simulink model "w13"  (R2025a)
settings: Solver=VariableStepAuto  StartTime=0.0  StopTime=3  FixedStep=1e-5  MaxStep=1e-4  RelTol=1e-3
values from neighbouring files (symbols this model uses):
  B = 0.0001    [main.m]
  Is_rated = 10    [main.m]
  J = 0.045    [main.m]
  Kas = 1/Kps    (= 3.05577490736)    [main.m]
  Kic = Rs*Wcc    (= 1256.63706144)    [main.m]
  Kis = J*Wsc^2/5/Kt    (= 2.05616758356)    [main.m]
  Kpc = Lds*Wcc    (= 18.8495559215)    [main.m]
  Kps = J*Wsc/Kt    (= 0.327249234749)    [main.m]
  Lamf = 0.12    [main.m]
  Lds = 30.0e-3    (= 0.03)    [main.m]
  Lqs = 40.0e-3    (= 0.04)    [main.m]
  P = 24    [main.m]
  Rs = 2    [main.m]
  Wcc = 100*2*pi    (= 628.318530718)    [main.m]
settings Model: Creator=moon  LastModifiedBy=New
settings RTWCC: GPUComputeCapability=3.5

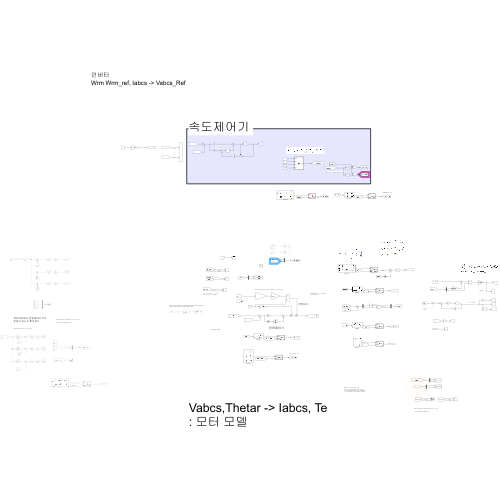
[thumbnail: Simulink's stored preview of the top-level diagram]
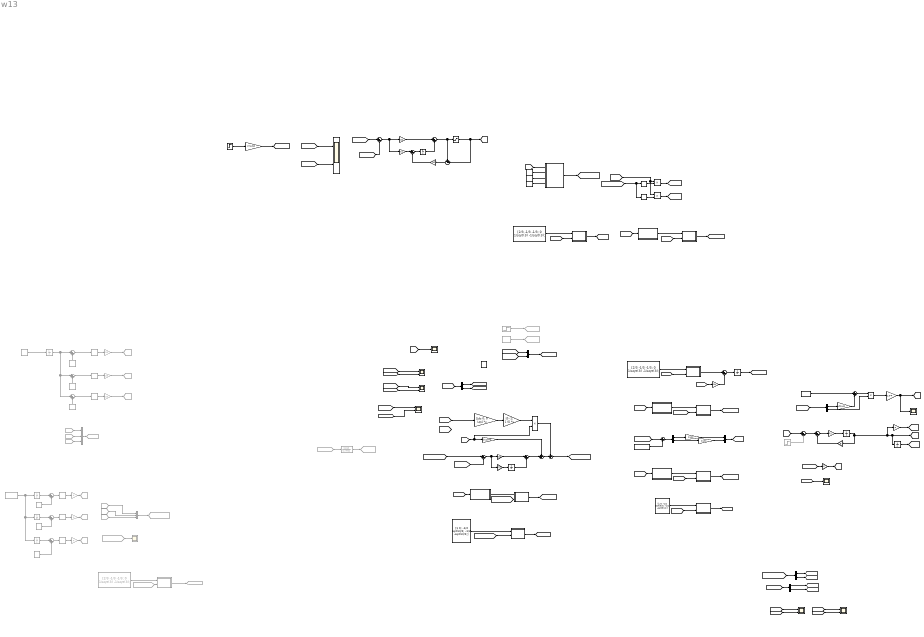
== system w13 ==
  note: 30도 더하면 속도제어가 안정적이게 된다
  note: E = w*phi 라서 속도는 전압에 비례
      | T는 전류에 비례
  note: 인버터
      | Wrm Wrm_ref, Iabcs -> Vabcs_Ref
  note: 전류제어기
  note: Vabcs,Thetar -> Iabcs, Te
      | : 모터 모델
  note: 컴퓨터에서 사용하는 값. 센싱된것. Idqsr과 무슨 차이? 센싱만?
  note: 센싱된 것을 사용해야
  note: 여기 수정함
  note: 여기서 부터는 모터
  note: 두개를 비교해보면 똑같을 것. 실제에 LPF를 넣을 순없다. LPF는 이상적인 상황. 이론적으로 실제 전류는 LPF와 이론적으로 같을 것이다
  note: feedback 이라는 뜻
  note: 속도제어기
  note: +였나?
  note: 전향보상
  note: 4Nm 만큼 거리가 발생해서 회전,
      | 외부 토크가 발생해도iqs 만큼 무조건 제어
      | 그럼 어떻게 회전자계와 회전자의 위치를 맞춰?
      | -> 기계 모델링을 무시: 대신 "wrm이 고정이다"
  note: d축과 q축 에 대한 정보가 아무 것도 없다
  note: 그래서 동기좌표 제어를 해야한다
  note: Wcc 와 We의 차이 만큼 딜레이와 크기 차이가 발생
  note: 정지좌표에서 전류제어기 무슨 문제가 있는지 확인한다
  note: 1/2 해야?
  note: Wcc 와 We의 차이 만큼 딜레이와 크기 차이가 발생
  note: 그래서 동기좌표 제어를 해야한다
  Constant : Constant  Commented=on  Value=10
  Constant1 : Constant  Commented=on  Value=2*pi/3
  Constant10 : Constant  Commented=on  Value=4
  Constant11 : Constant  Commented=on  Value=-4*pi/3
  Constant13 : Constant  Value=Lds
  Constant14 : Constant  Value=Lqs
  Constant15 : Constant  Value=Lamf
  Constant2 : Constant  Commented=on  Value=-2*pi/3
  Constant3 : Constant  Value=[Lamf 0 ]
  Constant4 : Constant  Value=Lamf
  Constant5 : Constant  Commented=on  Value=0
  Constant6 : Constant  Commented=on  Value=10*2*pi
  Constant7 : Constant  Commented=on  Value=0
  Constant8 : Constant  Value=0
  Constant9 : Constant  Commented=on  Value=-2*pi/3
  Cos : Trigonometry  Commented=on  Operator=cos
  Cos1 : Trigonometry  Commented=on  Operator=cos
  Cos2 : Trigonometry  Commented=on  Operator=cos
  Cos3 : Trigonometry  Operator=cos
  Demux{,1..2,4..5} (5 alike) : Demux  Outputs=2
  From18 : From  Commented=on  GotoTag=Vas
  From19 : From  Commented=on  GotoTag=Vbs
  From2 : From  Commented=on  GotoTag=Iabcs_Ref
  From20 : From  Commented=on  GotoTag=Vcs
  From22 : From  Commented=on  GotoTag=Ias_Ref
  From23 : From  Commented=on  GotoTag=Ibs_Ref
  From24 : From  Commented=on  GotoTag=Ics_Ref
  From26 : From  Commented=on  GotoTag=Iabcs_Ref
  From53 : From  Commented=on  GotoTag=Idqsr_Ref
  Gain : Gain  Commented=on  Gain=20
  Gain1 : Gain  Commented=on  Gain=20
  Gain10 : Gain  Gain=1/Lds
  Gain11 : Gain  Gain=1/Lqs
  Gain12 : Gain  Gain=[0 Lamf]
  Gain13 : Gain  Gain=[Lds 0; 0 Lqs]  Multiplication=Matrix(K*u)
  Gain14 : Gain  Gain=Kps
  Gain15 : Gain  Gain=Kis
  Gain16 : Gain  Gain=Kas
  Gain17 : Gain  Gain=2*pi/60
  Gain19 : Gain  Gain=Lds-Lqs
  Gain2 : Gain  Commented=on  Gain=20
  Gain20 : Gain  Gain=1.5*P
  Gain21 : Gain  Gain=Rs
  Gain22 : Gain  Gain=P
  Gain23 : Gain  Gain=1/J
  Gain24 : Gain  Gain=B
  Gain3 : Gain  Commented=on  Gain=4
  Gain4 : Gain  Commented=on  Gain=4
  Gain5 : Gain  Commented=on  Gain=4
  Gain6 : Gain  Gain=Kpc
  Gain7 : Gain  Gain=Kic
  Gain8 : Gain  Gain=[0 -1; 1 0]  Multiplication=Matrix(K*u)
  Gain9 : Gain  Gain=P
  Goto : Goto  Commented=on  GotoTag=Vas
  Goto1 : Goto  Commented=on  GotoTag=Vbs
  Goto14 : Goto  Commented=on  GotoTag=Ibs_Ref
  Goto15 : Goto  Commented=on  GotoTag=Ics_Ref
  Goto16 : Goto  Commented=on  GotoTag=Iabcs_Ref
  Goto17 : Goto  Commented=on  GotoTag=Idqss_Ref
  Goto18 : Goto  Commented=on  GotoTag=Idsr_Ref
  Goto19 : Goto  Commented=on  GotoTag=Iqsr_Ref
  Goto2 : Goto  Commented=on  GotoTag=Vcs
  Goto38 : Goto  Commented=on  GotoTag=Idqsr_FB
  Goto4 : Goto  Commented=on  GotoTag=Vabcs
  Goto9 : Goto  Commented=on  GotoTag=Ias_Ref
  Integrator{,4..6} (4 alike) : Integrator  Commented=on
  Integrator{1..3,7..8} (5 alike) : Integrator
  MATLAB Function : MATLAB Function  TreatAsAtomicUnit=on
  MATLAB Function1 : MATLAB Function  TreatAsAtomicUnit=on
  MATLAB Function2 : MATLAB Function  TreatAsAtomicUnit=on
  MATLAB Function3 : MATLAB Function  TreatAsAtomicUnit=on
  MATLAB Function4 : MATLAB Function  Commented=on  TreatAsAtomicUnit=on
  MATLAB Function5 : MATLAB Function  TreatAsAtomicUnit=on
  MATLAB Function6 : MATLAB Function  TreatAsAtomicUnit=on
  MATLAB Function7 : MATLAB Function  TreatAsAtomicUnit=on
  MATLAB Function8 : MATLAB Function  TreatAsAtomicUnit=on
  MATLAB Function9 : MATLAB Function  TreatAsAtomicUnit=on
  Mux : Mux  Commented=on  Inputs=3
  Mux1 : Mux  Commented=on  Inputs=3
  Mux2 : Mux  Inputs=2
  Mux3 : Mux  Inputs=2
  Product{,1..2,8} (4 alike) : Product
  R(-theta) : Subsystem
      mask Display: image(imread('img/rotateInverseMatrix.png'))
  R(-theta)1 : Subsystem
      mask Display: image(imread('img/rotateInverseMatrix.png'))
  R(theta) : Subsystem
      mask Display: image(imread('img/rotateMatrix.png'))
  R(theta)1 : Subsystem
      mask Display: image(imread('img/rotateMatrix.png'))
  Saturation : Saturate  UpperLimit=Is_rated  LowerLimit=-Is_rated
  Scope : Scope
      settings: ActiveDisplayYMinimum=-12.65498  ActiveDisplayYMaximum=12.66704
  Scope1 : Scope  Commented=on
      settings: ActiveDisplayYMinimum=-5  ActiveDisplayYMaximum=5
  Scope2 : Scope
      settings: ActiveDisplayYMinimum=-30.63126  ActiveDisplayYMaximum=63.40805  DataLoggingVariableName=ScopeData2
  Scope{3..8} (6 alike) : Scope  NumInputPorts=2
      Scope3 settings: ActiveDisplayYMinimum=-5.30172  ActiveDisplayYMaximum=0.86593  DataLoggingVariableName=ScopeData4
      Scope4 settings: ActiveDisplayYMinimum=-5.10751  ActiveDisplayYMaximum=5.1663  DataLoggingVariableName=ScopeData2
      Scope5 settings: ActiveDisplayYMinimum=-5.08231  ActiveDisplayYMaximum=5.15483  DataLoggingVariableName=ScopeData3
      Scope6 settings: ActiveDisplayYMinimum=-0.50888  ActiveDisplayYMaximum=4.57994  DataLoggingVariableName=ScopeData5
      Scope7 settings: ActiveDisplayYMinimum=-5.25048  ActiveDisplayYMaximum=7.25433  DataLoggingVariableName=ScopeData6
      Scope8 settings: ActiveDisplayYMinimum=-64.34522  ActiveDisplayYMaximum=579.10702
  Scope9 : Scope
      settings: ActiveDisplayYMinimum=-12.65498  ActiveDisplayYMaximum=12.66704
  Sin : Trigonometry  Commented=on
  Sin1 : Trigonometry  Commented=on
  Sin2 : Trigonometry  Commented=on
  Sin3 : Trigonometry
  Step : Step  After=4000  SampleTime=0
  Sum{,1..2,8..10} (6 alike) : Sum  Commented=on  Inputs=|++
  Sum{3..4,6..7,11,15,17} (7 alike) : Sum  Inputs=|+-
  Sum12 : Sum  Inputs=|++
  Sum13 : Sum  Inputs=++|
  Sum14 : Sum  Inputs=++|
  Sum16 : Sum  Inputs=|++
  Sum18 : Sum  Inputs=+-|
  Sum5 : Sum  Inputs=|++
  TL : Step  Commented=on  Time=0.5  SampleTime=0
  Transfer Fcn : TransferFcn  Commented=on  Numerator=[Wcc]  Denominator=[1 Wcc]
  abc to dq : Constant  Value=[2/3 -1/3 -1/3; 0 1/sqrt(3) -1/sqrt(3);]
      mask Display: image(imread('img/abc2dq.png'))
  abc to dq1 : Constant  Commented=on  Value=[2/3 -1/3 -1/3; 0 1/sqrt(3) -1/sqrt(3);]
      mask Display: image(imread('img/abc2dq.png'))
  abc to dq2 : Constant  Value=[2/3 -1/3 -1/3; 0 1/sqrt(3) -1/sqrt(3);]
      mask Display: image(imread('img/abc2dq.png'))
  "at 2s , 4A" : Step  Commented=on  Time=2  After=4  SampleTime=0
  dq to abc : Constant  Value=[1 0; -1/2 sqrt(3)/2; -1/2 -sqrt(3)/2;]
      mask Display: image(imread('img/dq2abc.png'))
  dq to abc1 : Constant  Value=[1 0; -1/2 sqrt(3)/2; -1/2 -sqrt(3)/2;]
      mask Display: image(imread('img/dq2abc.png'))
  wires:
  Gain/1 -> Goto/1
  Sin/1 -> Gain/1
  Sum/1 -> Sin/1
  Constant/1 -> Integrator/1  "angluar velocity"
  Sin1/1 -> Gain1/1
  Gain1/1 -> Goto1/1
  Sum1/1 -> Sin1/1
  Gain2/1 -> Goto2/1
  Sum2/1 -> Sin2/1
  Sin2/1 -> Gain2/1
  Integrator/1 -> Sum2/1, Sum1/1, Sum/1  "angle"
  Constant1/1 -> Sum1/2
  Constant2/1 -> Sum2/2
  Sum3/1 -> Integrator1/1
  Integrator1/1 -> [Lamdqss]
  MATLAB Function3/1(output) -> Sum3/1  "Vdqss"
  [Lamdqsr] -> Sum4/1
  Constant3/1 -> Sum4/2
  Sum4/1 -> Demux1/1
  Demux1/1 -> Gain10/1
  Demux1/2 -> Gain11/1
  Gain10/1 -> Mux2/1
  Gain11/1 -> Mux2/2
  Mux2/1 -> [Idqsr]
  [Idqsr] -> Demux4/1
  Demux4/1 -> Gain19/1
  Constant4/1 -> Sum5/1
  Gain19/1 -> Sum5/2
  Sum5/1 -> Product8/1
  Demux4/2 -> Product8/2
  Product8/1 -> Gain20/1
  Gain20/1 -> Scope2/1, [Te]
  [Te] -> Sum6/1
  Sum6/1 -> Sum7/1
  Integrator3/1 -> Gain24/1, Gain9/1, Integrator2/1, [Wrm]
  TL/1 -> Sum6/2
  [Idqss] -> Gain21/1
  Gain21/1 -> Sum3/2
  Gain22/1 -> [Thetar]
  [Thetarm] -> Gain22/1
  Integrator2/1 -> [Thetarm]
  Sum7/1 -> Gain23/1
  Gain23/1 -> Integrator3/1
  Gain24/1 -> Sum7/2
  dq to abc/1 -> MATLAB Function/1(input1)
  [Idqss] -> MATLAB Function/2(input2)
  MATLAB Function/1(output) -> [Iabcs]
  [Lamdqss] -> MATLAB Function1/2(input2)
  MATLAB Function1/1(output) -> [Lamdqsr]
  [Thetar] -> R(-theta)/1(t)
  R(-theta)/1(y) -> MATLAB Function1/1(input1)
  MATLAB Function2/1(output) -> [Idqss]
  [Thetar] -> R(theta)/1(t)
  R(theta)/1(y) -> MATLAB Function2/1(input1)
  [Idqsr] -> MATLAB Function2/2(input2)
  abc to dq/1 -> MATLAB Function3/1(input1)
  [Vabcs] -> MATLAB Function3/2(input2)
  From18/1 -> Mux1/1
  From19/1 -> Mux1/2
  From20/1 -> Mux1/3
  Mux1/1 -> Goto4/1
  [Iabcs] -> Scope/1
  Constant5/1 -> Sum/2
  Cos/1 -> Gain3/1
  Integrator4/1 -> Sum8/1  "angle"
  Constant7/1 -> Sum8/2
  Sum8/1 -> Cos/1
  Gain3/1 -> Goto9/1
  Gain4/1 -> Goto14/1
  Constant9/1 -> Sum9/2
  Integrator5/1 -> Sum9/1  "angle"
  Sum9/1 -> Cos1/1
  Cos1/1 -> Gain4/1
  Gain5/1 -> Goto15/1
  Constant11/1 -> Sum10/2
  Integrator6/1 -> Sum10/1  "angle"
  Sum10/1 -> Cos2/1
  Cos2/1 -> Gain5/1
  Constant6/1 -> Integrator6/1, Integrator5/1, Integrator4/1  "angluar velocity"
  From22/1 -> Mux/1
  From23/1 -> Mux/2
  From24/1 -> Mux/3
  Mux/1 -> Goto16/1
  MATLAB Function4/1(output) -> Goto17/1
  abc to dq1/1 -> MATLAB Function4/1(input1)
  From26/1 -> MATLAB Function4/2(input2)
  Gain6/1 -> Sum12/1
  Sum11/1 -> Gain7/1, Gain6/1
  Gain7/1 -> Integrator7/1
  Integrator7/1 -> Sum12/2
  dq to abc1/1 -> MATLAB Function5/1(input1)
  MATLAB Function5/1(output) -> [Vabcs]
  [Vdqss_Ref] -> MATLAB Function5/2(input2)
  Demux2/2 -> [Iqs_Ref]
  Demux2/1 -> [Ids_Ref]
  [Idqss_Ref] -> Demux2/1
  [Idqss] -> Demux5/1
  Demux5/1 -> [Idss]
  Demux5/2 -> [Iqss]
  [Ids_Ref] -> Scope4/1  "Ids_Ref"
  [Idss] -> Scope4/2  "Ids"
  [Iqss] -> Scope5/2  "Iqs"
  [Iqs_Ref] -> Scope5/1  "Iqs_Ref"
  From2/1 -> Scope1/1
  "at 2s , 4A"/1 -> Goto18/1
  Constant10/1 -> Goto19/1
  [Iqsr_Ref] -> Mux3/2
  [Idsr_Ref] -> Mux3/1
  Mux3/1 -> [Idqsr_Ref]
  MATLAB Function6/1(output) -> [Vdqss_Ref]
  R(theta)1/1(y) -> MATLAB Function6/1(input1)
  [Vdqsr_Ref] -> MATLAB Function6/2(input2)
  [Thetar] -> R(theta)1/1(t)
  [Idqsr] -> Demux/1
  Demux/2 -> [Iqsr]
  Demux/1 -> [Idsr]
  [Idsr_Ref] -> Scope3/1  "Idsr_Ref"
  [Idsr] -> Scope3/2  "Idsr"
  [Iqsr] -> Scope6/2
  [Iqsr_Ref] -> Scope6/1
  Sum12/1 -> Sum13/2
  Gain9/1 -> [Wr]
  [Wr] -> Product/2, Gain12/1
  Gain12/1 -> Sum13/1
  Sum13/1 -> Sum14/2
  Sum14/1 -> [Vdqsr_Ref]
  [Idqsr] -> Gain13/1
  Gain13/1 -> Gain8/1
  Gain8/1 -> Product/1
  Product/1 -> Sum14/1
  [Idqsr_Ref] -> Scope7/1  "Idqsr_Ref"
  [Idqsr] -> Scope7/2  "Idqsr"
  [Wrm_Ref] -> Sum15/1
  [Wrm] -> Sum15/2
  Gain14/1 -> Sum16/1
  Integrator8/1 -> Sum16/2
  Sum15/1 -> Gain15/1, Gain14/1
  Gain15/1 -> Sum17/1
  Sum17/1 -> Integrator8/1
  Sum16/1 -> Saturation/1, Sum18/1
  Saturation/1 -> [Is_Ref], Sum18/2
  Sum18/1 -> Gain16/1
  Gain16/1 -> Sum17/2
  [Is_Ref] -> MATLAB Function7/1(Is_Ref)
  Constant15/1 -> MATLAB Function7/4(Lamf)
  Constant14/1 -> MATLAB Function7/3(Lqs)
  Constant13/1 -> MATLAB Function7/2(Lds)
  MATLAB Function7/1(beta) -> [bate_opt]
  [bate_opt] -> Sin3/1, Cos3/1
  Cos3/1 -> Product1/2
  [Is_Ref] -> Product2/1, Product1/1
  Sin3/1 -> Product2/2
  Product2/1 -> [Iqsr_Ref]
  Product1/1 -> [Idsr_Ref]
  [Iabcs] -> MATLAB Function8/2(input2)
  abc to dq2/1 -> MATLAB Function8/1(input1)
  MATLAB Function8/1(output) -> [Idqss_FB]  "Vdqss"
  MATLAB Function9/1(output) -> [Idqsr_FB]
  R(-theta)1/1(y) -> MATLAB Function9/1(input1)
  [Idqss_FB] -> MATLAB Function9/2(input2)
  [Thetar] -> R(-theta)1/1(t)
  From53/1 -> Transfer Fcn/1
  Transfer Fcn/1 -> Goto38/1
  [Wrm_Ref] -> Scope8/1  "wrm_ref"
  [Wrm] -> Scope8/2  "wrm"
  Gain17/1 -> [Wrm_Ref]
  Step/1 -> Gain17/1
  [Idqsr_Ref] -> Sum11/1
  [Idqsr_FB] -> Sum11/2
  [Iabcs] -> Scope9/1

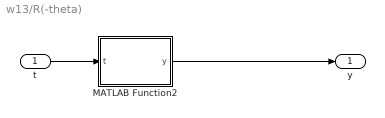
== system w13/R(-theta) ==
  t : Inport
  MATLAB Function2 : MATLAB Function  TreatAsAtomicUnit=on
  y : Outport
  wires:
  MATLAB Function2/1(y) -> y/1
  t/1 -> MATLAB Function2/1(t)

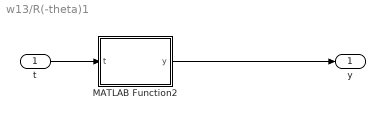
== system w13/R(-theta)1 ==
  t : Inport
  MATLAB Function2 : MATLAB Function  TreatAsAtomicUnit=on
  y : Outport
  wires:
  MATLAB Function2/1(y) -> y/1
  t/1 -> MATLAB Function2/1(t)

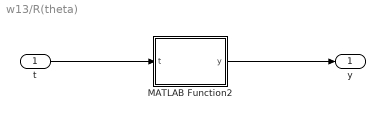
== system w13/R(theta) ==
  t : Inport
  MATLAB Function2 : MATLAB Function  TreatAsAtomicUnit=on
  y : Outport
  wires:
  MATLAB Function2/1(y) -> y/1
  t/1 -> MATLAB Function2/1(t)

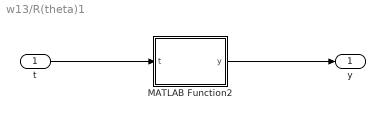
== system w13/R(theta)1 ==
  t : Inport
  MATLAB Function2 : MATLAB Function  TreatAsAtomicUnit=on
  y : Outport
  wires:
  MATLAB Function2/1(y) -> y/1
  t/1 -> MATLAB Function2/1(t)

== matlab function w13/MATLAB Function1 ==
  data: input1 input; output output; input2 input
function output = matrix_multiply(input1, input2)
    % 행렬 곱셈 (input1의 열 수 = input2의 행 수)
    output = input1 * input2;
end

== matlab function w13/MATLAB Function9 ==
  data: input1 input; output output; input2 input
function output = matrix_multiply(input1, input2)
    % 행렬 곱셈 (input1의 열 수 = input2의 행 수)
    output = input1 * input2;
end

== matlab function w13/R(-theta)1/MATLAB Function2 ==
  data: t input; y output
function y = matrix_output(t)
y = [cos(t) sin(t); -sin(t) cos(t)];

== matlab function w13/MATLAB Function ==
  data: input1 input; output output; input2 input
function output = matrix_multiply(input1, input2)
    % 행렬 곱셈 (input1의 열 수 = input2의 행 수)
    output = input1 * input2;
end

== matlab function w13/R(-theta)/MATLAB Function2 ==
  data: t input; y output
function y = matrix_output(t)
y = [cos(t) sin(t); -sin(t) cos(t)];

== matlab function w13/MATLAB Function2 ==
  data: input1 input; output output; input2 input
function output = matrix_multiply(input1, input2)
    % 행렬 곱셈 (input1의 열 수 = input2의 행 수)
    output = input1 * input2;
end

== matlab function w13/R(theta)/MATLAB Function2 ==
  data: t input; y output
function y = matrix_output(t)
y = [cos(t) -sin(t); sin(t) cos(t)];

== matlab function w13/MATLAB Function3 ==
  data: input1 input; output output; input2 input
function output = matrix_multiply(input1, input2)
    % 행렬 곱셈 (input1의 열 수 = input2의 행 수)
    output = input1 * input2;
end

== matlab function w13/MATLAB Function4 ==
  data: input1 input; output output; input2 input
function output = matrix_multiply(input1, input2)
    % 행렬 곱셈 (input1의 열 수 = input2의 행 수)
    output = input1 * input2;
end

== matlab function w13/MATLAB Function5 ==
  data: input1 input; output output; input2 input
function output = matrix_multiply(input1, input2)
    % 행렬 곱셈 (input1의 열 수 = input2의 행 수)
    output = input1 * input2;
end

== matlab function w13/MATLAB Function6 ==
  data: input1 input; output output; input2 input
function output = matrix_multiply(input1, input2)
    % 행렬 곱셈 (input1의 열 수 = input2의 행 수)
    output = input1 * input2;
end

== matlab function w13/R(theta)1/MATLAB Function2 ==
  data: t input; y output
function y = matrix_output(t)
y = [cos(t) -sin(t); sin(t) cos(t)];

== matlab function w13/MATLAB Function7 ==
  data: Is_Ref input; beta output; Lds input; Lqs input; Lamf input
function beta = fcn(Is_Ref, Lds, Lqs, Lamf)

beta = acos((-Lamf+sqrt(Lamf^2+8*(Lds-Lqs)^2*Is_Ref^2))/(4*(Lds-Lqs)*(Is_Ref+0.001)));

== matlab function w13/MATLAB Function8 ==
  data: input1 input; output output; input2 input
function output = matrix_multiply(input1, input2)
    % 행렬 곱셈 (input1의 열 수 = input2의 행 수)
    output = input1 * input2;
end
